simulink model "modelo_c"  (R2026a)
settings: Solver=VariableStepAuto  StopTime=20
settings Model: Creator=honda  LastModifiedBy=honda

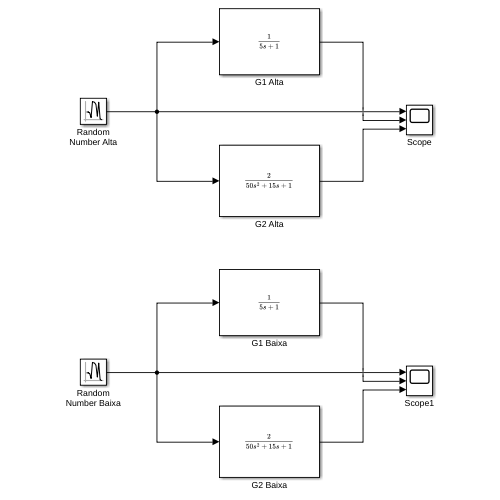
[thumbnail: Simulink's stored preview of the top-level diagram]
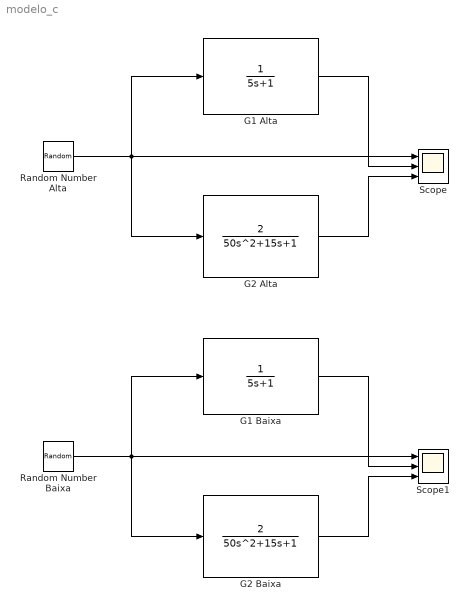
== system modelo_c ==
  G1 Alta : TransferFcn  Denominator=[5 1]
  G1 Baixa : TransferFcn  Denominator=[5 1]
  G2 Alta : TransferFcn  Numerator=[2]  Denominator=[50 15 1]
  G2 Baixa : TransferFcn  Numerator=[2]  Denominator=[50 15 1]
  Random Number Alta : RandomNumber  Variance=0.1  SampleTime=1
  Random Number Baixa : RandomNumber  Variance=0.001  SampleTime=1
  Scope : Scope  NumInputPorts=3
      settings: ActiveDisplayYMinimum=-0.585520043998924  ActiveDisplayYMaximum=0.696484444366221  DataLoggingVariableName=dados_c_alta
  Scope1 : Scope  NumInputPorts=3
      settings: ActiveDisplayYMinimum=-0.058552004399892395  ActiveDisplayYMaximum=0.069648444436622117  DataLoggingVariableName=dados_c_baixa
  wires:
  Random Number Alta/1 -> G1 Alta/1, Scope/1, G2 Alta/1
  G1 Alta/1 -> Scope/2
  G2 Alta/1 -> Scope/3
  Random Number Baixa/1 -> G1 Baixa/1, Scope1/1, G2 Baixa/1
  G2 Baixa/1 -> Scope1/3
  G1 Baixa/1 -> Scope1/2
